simulink model "simple_walk_3d_robot"  (R2015a)
settings: Solver=FixedStepDiscrete  StartTime=0.0  StopTime=inf  FixedStep=sample_time  RelTol=1e-3
InitFcn:
  | tg.sampletime = correctedSampleTime;
values from neighbouring files (symbols this model uses):
  sample_time = 1/sample_freq    (= 0.001)    [simulation_params.m]
settings Model: SimulationMode=external  CovSFcnEnable=off  Creator=wmartin  LastModifiedBy=robots
settings SolverCC: EnableConcurrentExecution=on
settings DataIOCC: LimitDataPoints=off  MaxDataPoints=1e7  SaveFormat=StructureWithTime  SignalLogging=off  DSMLogging=off
settings OptimizationCC: BlockReduction=off  OptimizeBlockIOStorage=off  BufferReuse=off  GlobalBufferReuse=off  ExpressionFolding=off  ExpressionDepthLimit=2147483647  LocalBlockOutputs=off  SimCompilerOptimization=on
settings DebuggingCC: UnderspecifiedInitializationDetection=Classic  MergeDetectMultiDrivingBlocksExec=none  SolverPrmCheckMsg=warning  StateNameClashWarn=warning
settings HardwareCC: ProdIntDivRoundTo=Zero  ProdEndianess=LittleEndian  ProdLongLongMode=on  ProdHWDeviceType=Generic->32-bit x86 compatible
settings ModelReferenceCC: UpdateModelReferenceTargets=IfOutOfDate  ModelReferenceNumInstancesAllowed=Single  ModelReferenceMinAlgLoopOccurrences=on
settings RTWCC: SystemTargetFile=slrt.tlc  TemplateMakefile=slrt_default_tmf  Description=Simulink Real-Time  RTWVerbose=off  RTWCompilerOptimization=on
settings CodeAppCC: MaxIdLength=256
settings SimulinkRealTimeCC: GeneratePreprocessorConditionals=Disable all  RL32LogBufSizeModifier=1e8

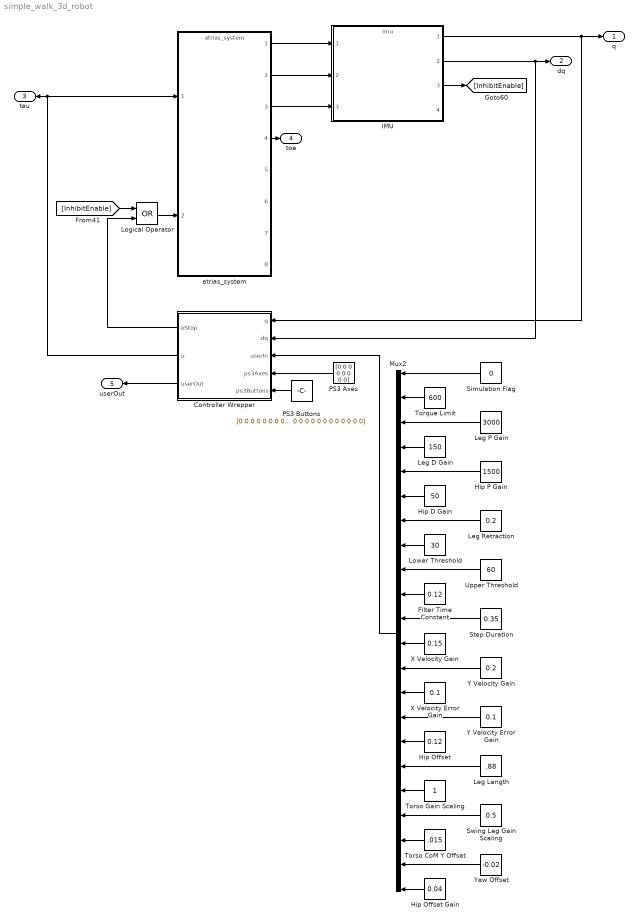
== system simple_walk_3d_robot ==
  Controller Wrapper : MATLAB Function  TreatAsAtomicUnit=on
  Filter Time Constant : Constant  Value=0.12  SampleTime=sample_time
  Hip D Gain : Constant  Value=50  SampleTime=sample_time
  Hip Offset : Constant  Value=0.12  SampleTime=sample_time
  Hip Offset Gain : Constant  Value=0.04  SampleTime=sample_time
  Hip P Gain : Constant  Value=1500  SampleTime=sample_time
  IMU : ModelReference  ModelNameDialog=imu  SimulationMode=Normal  ModelReferenceVersion=1.2451  CopyOfModelName=imu  DefaultDataLogging=on
  Leg D Gain : Constant  Value=150  SampleTime=sample_time
  Leg Length : Constant  Value=.88  SampleTime=sample_time
  Leg P Gain : Constant  Value=3000  SampleTime=sample_time
  Leg Retraction : Constant  Value=0.2  SampleTime=sample_time
  Logical Operator : Logic  Operator=OR  AllPortsSameDT=off  OutDataTypeStr=boolean
  Lower Threshold : Constant  Value=30  SampleTime=sample_time
  Mux2 : Mux  Inputs=22
  PS3 Axes : Constant  Value=[0 0 0 0 0 0 0 0]
  PS3 Buttons : Constant  Value=[0 0 0 0 0 0 0 0 0 0 0 0 0 0 0 0 0 0 0 0]
  Simulation Flag : Constant  Value=0  SampleTime=sample_time
  Step Duration : Constant  Value=0.35  SampleTime=sample_time
  Swing Leg Gain Scaling : Constant  Value=0.5  SampleTime=sample_time
  Torque Limit : Constant  Value=600  SampleTime=sample_time
  Torso CoM Y Offset : Constant  Value=.015  SampleTime=sample_time
  Torso Gain Scaling : Constant  SampleTime=sample_time
  Upper Threshold : Constant  Value=60  SampleTime=sample_time
  X Velocity Error Gain : Constant  Value=0.1  SampleTime=sample_time
  X Velocity Gain : Constant  Value=0.15  SampleTime=sample_time
  Y Velocity Error Gain : Constant  Value=0.1  SampleTime=sample_time
  Y Velocity Gain : Constant  Value=0.2  SampleTime=sample_time
  Yaw Offset : Constant  Value=-0.02  SampleTime=sample_time
  atrias_system : ModelReference  ModelNameDialog=atrias_system  SimulationMode=Normal  ModelReferenceVersion=1.2603  CopyOfModelName=atrias_system  DefaultDataLogging=on
  q : Outport
  dq : Outport  Port=2
  tau : Outport  Port=3
  toe : Outport  Port=4
  userOut : Outport  Port=5
  wires:
  Controller Wrapper/2(u) -> atrias_system/1, tau/1
  atrias_system/4 -> toe/1
  IMU/3 -> [InhibitEnable]
  Logical Operator/1 -> atrias_system/2
  [InhibitEnable] -> Logical Operator/1
  Controller Wrapper/1(eStop) -> Logical Operator/2
  IMU/1 -> Controller Wrapper/1(q), q/1
  IMU/2 -> Controller Wrapper/2(dq), dq/1
  atrias_system/1 -> IMU/1
  atrias_system/2 -> IMU/2
  atrias_system/3 -> IMU/3
  PS3 Axes/1 -> Controller Wrapper/4(ps3Axes)
  Controller Wrapper/3(userOut) -> userOut/1
  Mux2/1 -> Controller Wrapper/3(userIn)
  Torque Limit/1 -> Mux2/2
  Leg P Gain/1 -> Mux2/3
  Leg D Gain/1 -> Mux2/4
  Hip P Gain/1 -> Mux2/5
  Hip D Gain/1 -> Mux2/6
  Leg Retraction/1 -> Mux2/7
  Lower Threshold/1 -> Mux2/8
  Upper Threshold/1 -> Mux2/9
  Y Velocity Gain/1 -> Mux2/13
  X Velocity Gain/1 -> Mux2/12
  Step Duration/1 -> Mux2/11
  Filter Time Constant/1 -> Mux2/10
  Simulation Flag/1 -> Mux2/1
  X Velocity Error Gain/1 -> Mux2/14
  Y Velocity Error Gain/1 -> Mux2/15
  Hip Offset/1 -> Mux2/16
  Swing Leg Gain Scaling/1 -> Mux2/19
  Leg Length/1 -> Mux2/17
  Torso Gain Scaling/1 -> Mux2/18
  Torso CoM Y Offset/1 -> Mux2/20
  Yaw Offset/1 -> Mux2/21
  Hip Offset Gain/1 -> Mux2/22
  PS3 Buttons/1 -> Controller Wrapper/5(ps3Buttons)

== matlab function simple_walk_3d_robot/Controller Wrapper ==
  data: q input; dq input; userIn input; ps3Axes input; eStop output; u output; userOut output; ps3Buttons input
function [eStop, u, userOut] = wrapper(q, dq, userIn, ps3Axes, ps3Buttons)
%WRAPPER Controller wrapper.
%
% Notes:
% 	- State indexes (q and qdot)
%       (rBl rBm rAl rAm lBl lBm lAl lAm rHm lHm bR bY bP) 
%   - Input indexes (u)
%       (rB rA rH lB lA lH)
    
    % Actual controller function
    [eStop, u, userOut] = controller(q, dq, userIn, ps3Axes, ps3Buttons);
end % wrapper
